simulink model "dip_ut"  (R2013b)
settings: Solver=FixedStepDiscrete  StartTime=0.0  StopTime=Inf  FixedStep=0.005  RelTol=1e-3
PostLoadFcn:
  | , if any(exist('dsrtsu_mdlpostloadfcn', 'file') == [2, 3, 6]), try dsrtsu_mdlpostloadfcn('Execute', bdroot); catch fprintf('Error in PostLoadFcn (dsrtsu_mdlpostloadfcn) for model "%s":\n %s\n', bdroot, lasterr); end, end,
undefined symbols (not defined in the file or in its folder): VLFC_LFCActing_flg, VLFC_LFCState_enum, VPER_LeftLaneAvail_flg, VPER_NumberOfTargets_enum, VPER_RightLaneAvail_flg
libraries: siltestlib x14, dip x1, simulink x1
settings Model: DSRTSU_INTERNAL_RTI_VER=450  DSRTSU_INTERNAL_RTI_TYPE=rti1401  RTICANMMDATA=struct('GeneralSetupData',struct('modelroot','C:\ADAS\trunk\ADAS_Softwares\HTDragon\software\sw_development\arch\app\dip','generalsettings',struct('filesettings',struct('destfolder',struct('Name','RTICANMM_FILES','Check',1),'buildfolder',struct('Name','.','Check',1),'AbsDestfolder',struct('Name','C:\ADAS\trunk\ADAS_Softwares\HTDragon\software\sw_development\arch\app\dip\RTICANMM_FILES'),'AbsBuildfolder',struct('Name','C:\ADAS\trunk\ADAS_Softwares\HTDragon\software\sw_development\arch\app\dip'))),'options',struct('addpaths',1,'rmpaths',1,'addtrcexclusion',logical(1),'cannavigator',struct('checkmonitoring',0),'show_usrtrc',0,'use_usrtrc',0),'advanced',struct('options',[1 1 1 1 1 1 1 1 1 1 1 1 1 1 1 1 1 1 1 1 1 1 1 1 1 1 1 1 1 1 1 1 1 1 1 1 1 1 1 1 1 1 1 1 1 1 1 1 1 1 1 1 1 1 1 1 1 1 1 1 1 1 1 1 1 1 1 1 1 1 1 1 1 1 1 1 1 1 1 1 1 1 1 1 1 1 1 1 1 1 1 1 1 1 1 1 1 1 1 1]),'MPSetup',{{}},'modelname','dip_ut','block','dip_ut'))  DSRTSU_INTERNAL_RTIFPGA=40  BufferReuse=off  Creator=13192  LastModifiedBy=13192
settings OptimizationCC: BlockReduction=off  OptimizeBlockIOStorage=off  BufferReuse=off  ExpressionFolding=off  LocalBlockOutputs=off
settings HardwareCC: ProdIntDivRoundTo=Zero  ProdEndianess=BigEndian  ProdHWDeviceType=Generic->Custom  TargetIntDivRoundTo=Zero  TargetEndianess=BigEndian  TargetHWDeviceType=Generic->Custom
settings RTWCC: SystemTargetFile=rti1401.tlc  MakeCommand=make_rti  TemplateMakefile=rti1401.tmf  Description=dSPACE DS1401 Hardware Platform  ProcessScript=rti1401_make_rtw_hook
settings STFCustomTargetCC: ParMdlRefBuildCompliant=on  GeneratePreprocessorConditionals=Disable all  MatFileLogging=on  SystemTargetFile=rti1401.tlc
settings GRTTargetCC: CompOptLevelCompliant=off  ConcurrentExecutionCompliant=off  CombineOutputUpdateFcns=off  GRTInterface=on  ExtModeMexFile=noextcomm

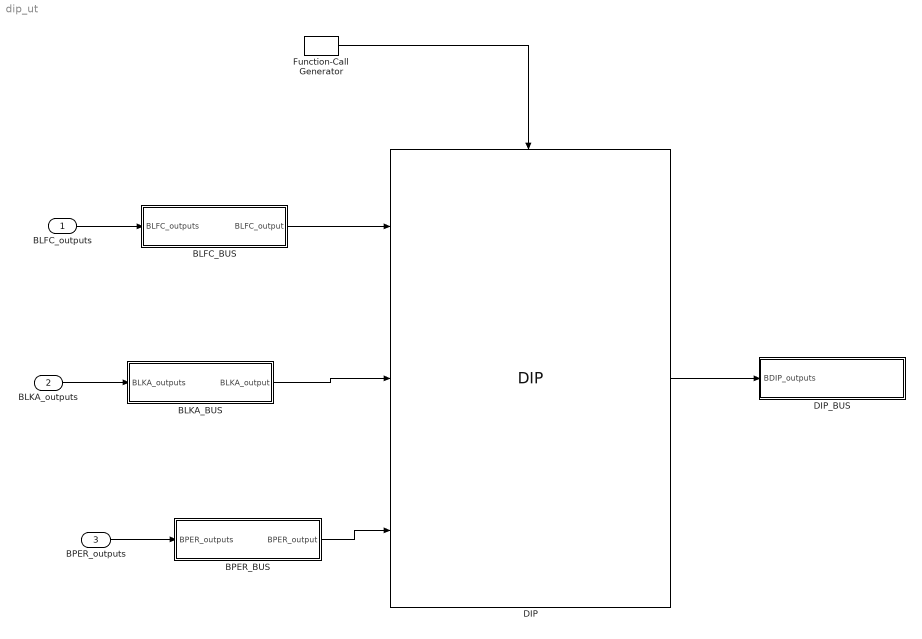
== system dip_ut ==
  BLFC_outputs : Inport  OutDataTypeStr=Bus: BLFC_outputs
  BLKA_outputs : Inport  Port=2  OutDataTypeStr=Bus: BLKA_outputs
  BPER_outputs : Inport  Port=3  OutDataTypeStr=Bus: BPER_outputs
  BLFC_BUS : Subsystem
  BLKA_BUS : Subsystem
  BPER_BUS : Subsystem
  DIP : dip/DIP
  DIP_BUS : Subsystem
  Function-Call Generator : simulink/Ports & Subsystems/Function-Call Generator  sample_time=0.005  numberOfIterations=1
  wires:
  BLFC_outputs/1 -> BLFC_BUS/1(BLFC_outputs)
  BLFC_BUS/1(BLFC_output) -> DIP/1
  BLKA_outputs/1 -> BLKA_BUS/1(BLKA_outputs)
  BLKA_BUS/1(BLKA_output) -> DIP/2
  BPER_outputs/1 -> BPER_BUS/1(BPER_outputs)
  BPER_BUS/1(BPER_output) -> DIP/3
  Function-Call Generator/1 -> DIP/Trigger
  DIP/1 -> DIP_BUS/1(BDIP_outputs)

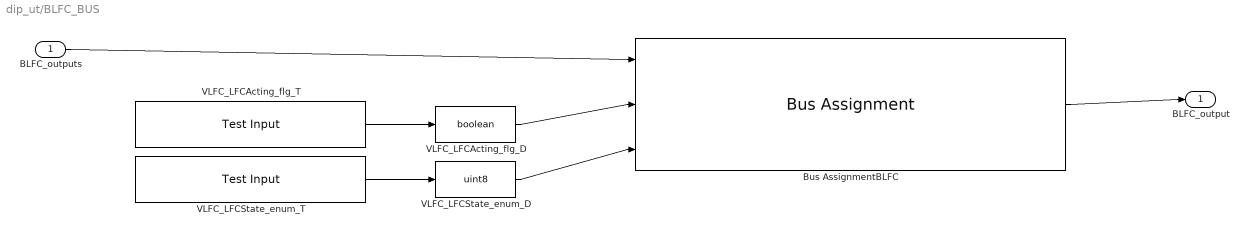
== system dip_ut/BLFC_BUS ==
  BLFC_outputs : Inport  OutDataTypeStr=Bus: BLFC_outputs
  Bus AssignmentBLFC : BusAssignment  AssignedSignals=VLFC_LFCActing_flg,VLFC_LFCState_enum
  VLFC_LFCActing_flg_D : DataTypeConversion  OutDataTypeStr=boolean
  VLFC_LFCActing_flg_T : siltestlib/Test Input  varname=VLFC_LFCActing_flg  sampletime=-1
  VLFC_LFCState_enum_D : DataTypeConversion  OutDataTypeStr=uint8
  VLFC_LFCState_enum_T : siltestlib/Test Input  varname=VLFC_LFCState_enum  sampletime=-1
  BLFC_output : Outport  OutDataTypeStr=Bus: BLFC_outputs
  wires:
  VLFC_LFCActing_flg_T/1 -> VLFC_LFCActing_flg_D/1
  VLFC_LFCState_enum_T/1 -> VLFC_LFCState_enum_D/1
  BLFC_outputs/1 -> Bus AssignmentBLFC/1
  Bus AssignmentBLFC/1 -> BLFC_output/1
  VLFC_LFCActing_flg_D/1 -> Bus AssignmentBLFC/2
  VLFC_LFCState_enum_D/1 -> Bus AssignmentBLFC/3

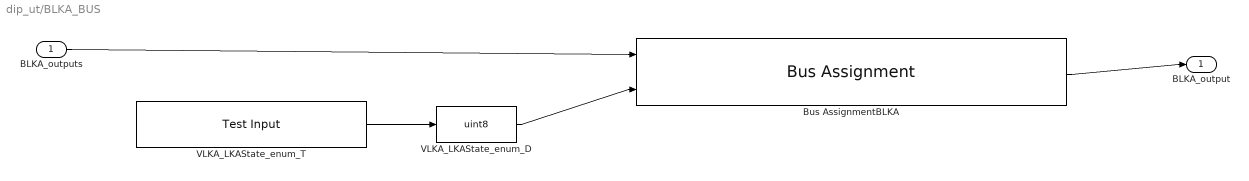
== system dip_ut/BLKA_BUS ==
  BLKA_outputs : Inport  OutDataTypeStr=Bus: BLKA_outputs
  Bus AssignmentBLKA : BusAssignment  AssignedSignals=VLKA_LKAState_enum
  VLKA_LKAState_enum_D : DataTypeConversion  OutDataTypeStr=uint8
  VLKA_LKAState_enum_T : siltestlib/Test Input  varname=VLKA_LKAState_enum  sampletime=-1
  BLKA_output : Outport  OutDataTypeStr=Bus: BLKA_outputs
  wires:
  VLKA_LKAState_enum_T/1 -> VLKA_LKAState_enum_D/1
  BLKA_outputs/1 -> Bus AssignmentBLKA/1
  Bus AssignmentBLKA/1 -> BLKA_output/1
  VLKA_LKAState_enum_D/1 -> Bus AssignmentBLKA/2

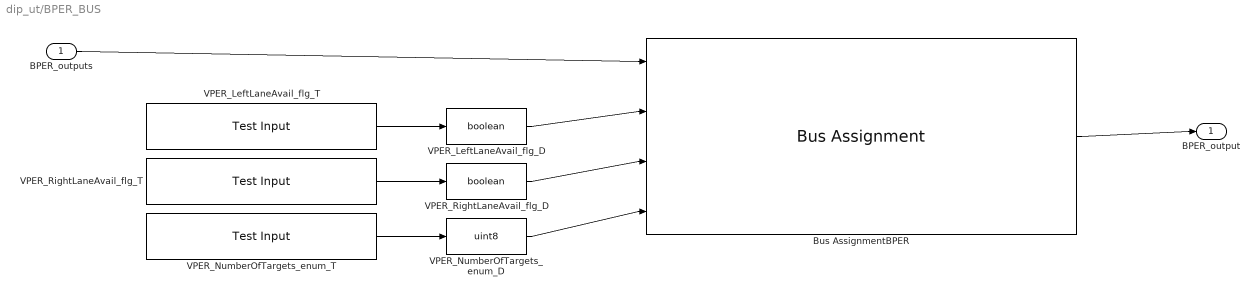
== system dip_ut/BPER_BUS ==
  BPER_outputs : Inport  OutDataTypeStr=Bus: BPER_outputs
  Bus AssignmentBPER : BusAssignment  AssignedSignals=VPER_LeftLaneAvail_flg,VPER_RightLaneAvail_flg,VPER_NumberOfTargets_enum
  VPER_LeftLaneAvail_flg_D : DataTypeConversion  OutDataTypeStr=boolean
  VPER_LeftLaneAvail_flg_T : siltestlib/Test Input  varname=VPER_LeftLaneAvail_flg  sampletime=-1
  VPER_NumberOfTargets_enum_D : DataTypeConversion  OutDataTypeStr=uint8
  VPER_NumberOfTargets_enum_T : siltestlib/Test Input  varname=VPER_NumberOfTargets_enum  sampletime=-1
  VPER_RightLaneAvail_flg_D : DataTypeConversion  OutDataTypeStr=boolean
  VPER_RightLaneAvail_flg_T : siltestlib/Test Input  varname=VPER_RightLaneAvail_flg  sampletime=-1
  BPER_output : Outport  OutDataTypeStr=Bus: BPER_outputs
  wires:
  VPER_LeftLaneAvail_flg_T/1 -> VPER_LeftLaneAvail_flg_D/1
  VPER_RightLaneAvail_flg_T/1 -> VPER_RightLaneAvail_flg_D/1
  VPER_NumberOfTargets_enum_T/1 -> VPER_NumberOfTargets_enum_D/1
  BPER_outputs/1 -> Bus AssignmentBPER/1
  Bus AssignmentBPER/1 -> BPER_output/1
  VPER_LeftLaneAvail_flg_D/1 -> Bus AssignmentBPER/2
  VPER_RightLaneAvail_flg_D/1 -> Bus AssignmentBPER/3
  VPER_NumberOfTargets_enum_D/1 -> Bus AssignmentBPER/4

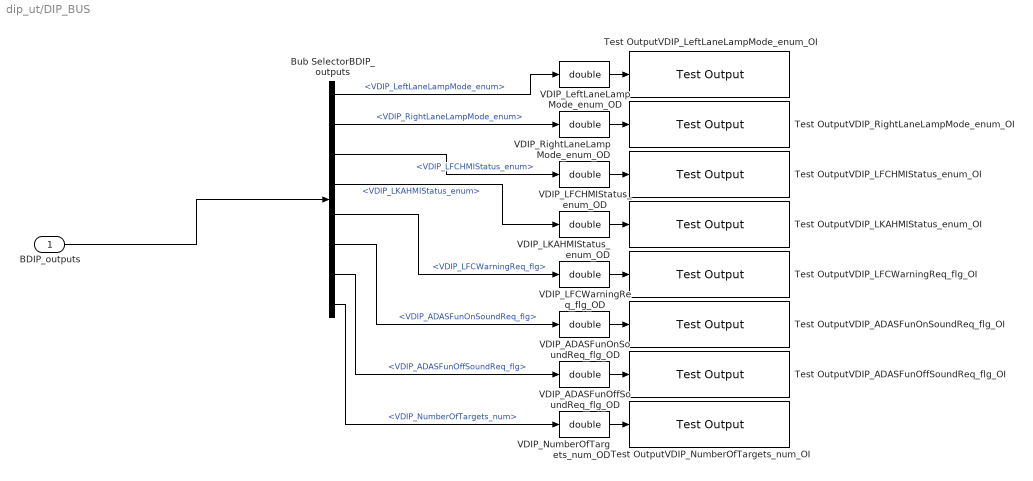
== system dip_ut/DIP_BUS ==
  BDIP_outputs : Inport  OutDataTypeStr=Bus: BDIP_outputs
  Bub SelectorBDIP_outputs : BusSelector  OutputSignals=VDIP_LeftLaneLampMode_enum,VDIP_RightLaneLampMode_enum,VDIP_LFCHMIStatus_enum,VDIP_LKAHMIStatus_enum,VDIP_LFCWarningReq_flg,VDIP_ADASFunOnSoundReq_flg,VDIP_ADASFunOffSoundReq_flg,VDIP_NumberOfTargets_num
  Test OutputVDIP_ADASFunOffSoundReq_flg_OI : siltestlib/Test Output  varname=VDIP_ADASFunOffSoundReq_flg  sampletime=-1
  Test OutputVDIP_ADASFunOnSoundReq_flg_OI : siltestlib/Test Output  varname=VDIP_ADASFunOnSoundReq_flg  sampletime=-1
  Test OutputVDIP_LFCHMIStatus_enum_OI : siltestlib/Test Output  varname=VDIP_LFCHMIStatus_enum  sampletime=-1
  Test OutputVDIP_LFCWarningReq_flg_OI : siltestlib/Test Output  varname=VDIP_LFCWarningReq_flg  sampletime=-1
  Test OutputVDIP_LKAHMIStatus_enum_OI : siltestlib/Test Output  varname=VDIP_LKAHMIStatus_enum  sampletime=-1
  Test OutputVDIP_LeftLaneLampMode_enum_OI : siltestlib/Test Output  varname=VDIP_LeftLaneLampMode_enum  sampletime=-1
  Test OutputVDIP_NumberOfTargets_num_OI : siltestlib/Test Output  varname=VDIP_NumberOfTargets_num  sampletime=-1
  Test OutputVDIP_RightLaneLampMode_enum_OI : siltestlib/Test Output  varname=VDIP_RightLaneLampMode_enum  sampletime=-1
  VDIP_ADASFunOffSoundReq_flg_OD : DataTypeConversion  OutDataTypeStr=double
  VDIP_ADASFunOnSoundReq_flg_OD : DataTypeConversion  OutDataTypeStr=double
  VDIP_LFCHMIStatus_enum_OD : DataTypeConversion  OutDataTypeStr=double
  VDIP_LFCWarningReq_flg_OD : DataTypeConversion  OutDataTypeStr=double
  VDIP_LKAHMIStatus_enum_OD : DataTypeConversion  OutDataTypeStr=double
  VDIP_LeftLaneLampMode_enum_OD : DataTypeConversion  OutDataTypeStr=double
  VDIP_NumberOfTargets_num_OD : DataTypeConversion  OutDataTypeStr=double
  VDIP_RightLaneLampMode_enum_OD : DataTypeConversion  OutDataTypeStr=double
  wires:
  VDIP_LeftLaneLampMode_enum_OD/1 -> Test OutputVDIP_LeftLaneLampMode_enum_OI/1
  VDIP_RightLaneLampMode_enum_OD/1 -> Test OutputVDIP_RightLaneLampMode_enum_OI/1
  VDIP_LFCHMIStatus_enum_OD/1 -> Test OutputVDIP_LFCHMIStatus_enum_OI/1
  VDIP_LKAHMIStatus_enum_OD/1 -> Test OutputVDIP_LKAHMIStatus_enum_OI/1
  VDIP_LFCWarningReq_flg_OD/1 -> Test OutputVDIP_LFCWarningReq_flg_OI/1
  VDIP_ADASFunOnSoundReq_flg_OD/1 -> Test OutputVDIP_ADASFunOnSoundReq_flg_OI/1
  VDIP_ADASFunOffSoundReq_flg_OD/1 -> Test OutputVDIP_ADASFunOffSoundReq_flg_OI/1
  VDIP_NumberOfTargets_num_OD/1 -> Test OutputVDIP_NumberOfTargets_num_OI/1
  BDIP_outputs/1 -> Bub SelectorBDIP_outputs/1
  Bub SelectorBDIP_outputs/1 -> VDIP_LeftLaneLampMode_enum_OD/1  "<VDIP_LeftLaneLampMode_enum>"
  Bub SelectorBDIP_outputs/2 -> VDIP_RightLaneLampMode_enum_OD/1  "<VDIP_RightLaneLampMode_enum>"
  Bub SelectorBDIP_outputs/3 -> VDIP_LFCHMIStatus_enum_OD/1  "<VDIP_LFCHMIStatus_enum>"
  Bub SelectorBDIP_outputs/4 -> VDIP_LKAHMIStatus_enum_OD/1  "<VDIP_LKAHMIStatus_enum>"
  Bub SelectorBDIP_outputs/5 -> VDIP_LFCWarningReq_flg_OD/1  "<VDIP_LFCWarningReq_flg>"
  Bub SelectorBDIP_outputs/6 -> VDIP_ADASFunOnSoundReq_flg_OD/1  "<VDIP_ADASFunOnSoundReq_flg>"
  Bub SelectorBDIP_outputs/7 -> VDIP_ADASFunOffSoundReq_flg_OD/1  "<VDIP_ADASFunOffSoundReq_flg>"
  Bub SelectorBDIP_outputs/8 -> VDIP_NumberOfTargets_num_OD/1  "<VDIP_NumberOfTargets_num>"
